simulink model "simRouteA_v4_11"  (R2015a)
settings: Solver=FixedStepDiscrete  StartTime=0.0  StopTime=36000  FixedStep=1  RelTol=1e-3
PreLoadFcn:
  | loadTimetable
StopFcn:
  | postProcess
undefined symbols (not defined in the file or in its folder): setBus1IntergenTime, setBus2IntergenTime, setBus3IntergenTime, setBus4IntergenTime
(part 2 of 7)

== system simRouteA_v4_11/Subsystem ==
  ID : Inport
  tTable : Inport  Port=2
  Constant12 : Constant  Value=10000
  Constant13 : Constant
  Direct Lookup Table (n-D)1 : LookupNDDirect  TableIsInput=on
  Divide1 : Product  Inputs=/*
  Math Function1 : Math  Operator=mod  SaturateOnIntegerOverflow=on
  Rounding : Rounding  Operator=round
  Rounding1 : Rounding  Operator=round
  Subtract1 : Sum  Inputs=-+
  schedTime : Outport
  wires:
  Rounding1/1 -> Direct Lookup Table (n-D)1/1
  Constant12/1 -> Math Function1/2, Divide1/1
  Constant13/1 -> Subtract1/1
  Divide1/1 -> Rounding/1
  Subtract1/1 -> Direct Lookup Table (n-D)1/2
  Direct Lookup Table (n-D)1/1 -> schedTime/1
  tTable/1 -> Direct Lookup Table (n-D)1/3
  Math Function1/1 -> Rounding1/1
  Rounding/1 -> Subtract1/2
  ID/1 -> Divide1/2, Math Function1/1

== system simRouteA_v4_11/Subsystem3 ==
  crnSched : Inport
  time : Inport  Port=2
  Constant2 : Constant  Value=0
  MinMax : MinMax  Function=max  Inputs=2
  Subtract1 : Sum  Inputs=+-
  tHoldCrnBus : Outport
  wires:
  time/1 -> Subtract1/2
  crnSched/1 -> Subtract1/1
  Subtract1/1 -> MinMax/1
  MinMax/1 -> tHoldCrnBus/1
  Constant2/1 -> MinMax/2

== system simRouteA_v4_11/atStopS1 ==
  paxDemandRate : Inport
  paxAlightRate : Inport  Port=2
  FIFO Queue9 : FIFOQueue
  busDwellThisStop : Subsystem
  calcPaxActivThisStop : Subsystem
  integrPaxAlightS1 : Subsystem
  integrPaxArrS1 : Subsystem
  setPaxAttribThisStop : SetAttribute  AttributeName=paxArr|paxAlight  AttributeFrom=Signal port|Signal port  AttributeValue=1|1  AttributeTreatAsVector=1|1  EvaluatedAttributeValue={ []; [] }
      settings: InputPortMap=u0,u1
  busIn : PMIOPort  Port=1  Side=Left
  busOut : PMIOPort  Port=2  Side=Right
  accPaxAlight : Outport
  accPaxDemand : Outport  Port=2
  crnVacancy : Outport  Port=3
  paxAlight : Outport  Port=4
  paxDemand : Outport  Port=5
  busIDAfterPaxCal : Outport  Port=6
  newVacancy : Outport  Port=7
  paxBoard : Outport  Port=8
  paxRemain : Outport  Port=9
  paxWait : Outport  Port=10
  intgPaxArr : Outport  Port=11
  intgPaxAlight : Outport  Port=12
  idBusLeave : Outport  Port=13
  wires:
  calcPaxActivThisStop/4(busID) -> busIDAfterPaxCal/1
  calcPaxActivThisStop/1(vacanIn) -> crnVacancy/1
  calcPaxActivThisStop/5(newVacan) -> newVacancy/1
  calcPaxActivThisStop/7(paxRemain) -> paxRemain/1
  paxAlightRate/1 -> integrPaxAlightS1/1(ratePax)
  calcPaxActivThisStop/3(paxArr) -> paxDemand/1
  busDwellThisStop/1(idBusLeave) -> idBusLeave/1
  calcPaxActivThisStop/6(paxBoard) -> paxBoard/1
  calcPaxActivThisStop/9(intgPaxArr) -> intgPaxArr/1
  calcPaxActivThisStop/8(paxWait) -> paxWait/1
  integrPaxArrS1/1(accPax) -> accPaxDemand/1, setPaxAttribThisStop/1
  integrPaxAlightS1/1(accPax) -> accPaxAlight/1, setPaxAttribThisStop/2
  calcPaxActivThisStop/11(dwellTime) -> busDwellThisStop/1(dwellTime)
  calcPaxActivThisStop/10(intgPaxAlight) -> intgPaxAlight/1
  calcPaxActivThisStop/2(paxAlight) -> paxAlight/1
  paxDemandRate/1 -> integrPaxArrS1/1(ratePax)
  connections:
  FIFO Queue9/LConn1 -- busIn/RConn1
  busDwellThisStop/RConn1 -- busOut/RConn1
  setPaxAttribThisStop/RConn1 -- calcPaxActivThisStop/LConn1
  FIFO Queue9/RConn1 -- setPaxAttribThisStop/LConn1
  busDwellThisStop/LConn1 -- calcPaxActivThisStop/RConn1

== system simRouteA_v4_11/atStopS10 ==
  paxDemandRate : Inport
  paxAlightRate : Inport  Port=2
  FIFO Queue9 : FIFOQueue
  busDwellThisStop : Subsystem
  calcPaxActivThisStop : Subsystem
  integrPaxAlightS1 : Subsystem
  integrPaxArrS1 : Subsystem
  setPaxAttribThisStop : SetAttribute  AttributeName=paxArr|paxAlight  AttributeFrom=Signal port|Signal port  AttributeValue=1|1  AttributeTreatAsVector=1|1  EvaluatedAttributeValue={ []; [] }
      settings: InputPortMap=u0,u1
  busIn : PMIOPort  Port=1  Side=Left
  busOut : PMIOPort  Port=2  Side=Right
  accPaxAlight : Outport
  accPaxDemand : Outport  Port=2
  crnVacancy : Outport  Port=3
  paxAlight : Outport  Port=4
  paxDemand : Outport  Port=5
  busIDAfterPaxCal : Outport  Port=6
  newVacancy : Outport  Port=7
  paxBoard : Outport  Port=8
  paxRemain : Outport  Port=9
  paxWait : Outport  Port=10
  intgPaxArr : Outport  Port=11
  intgPaxAlight : Outport  Port=12
  idBusLeave : Outport  Port=13
  wires:
  calcPaxActivThisStop/4(busID) -> busIDAfterPaxCal/1
  calcPaxActivThisStop/1(vacanIn) -> crnVacancy/1
  calcPaxActivThisStop/5(newVacan) -> newVacancy/1
  calcPaxActivThisStop/7(paxRemain) -> paxRemain/1
  paxAlightRate/1 -> integrPaxAlightS1/1(ratePax)
  calcPaxActivThisStop/3(paxArr) -> paxDemand/1
  busDwellThisStop/1(idBusLeave) -> idBusLeave/1
  calcPaxActivThisStop/6(paxBoard) -> paxBoard/1
  calcPaxActivThisStop/9(intgPaxArr) -> intgPaxArr/1
  calcPaxActivThisStop/8(paxWait) -> paxWait/1
  integrPaxArrS1/1(accPax) -> accPaxDemand/1, setPaxAttribThisStop/1
  integrPaxAlightS1/1(accPax) -> accPaxAlight/1, setPaxAttribThisStop/2
  calcPaxActivThisStop/11(dwellTime) -> busDwellThisStop/1(dwellTime)
  calcPaxActivThisStop/10(intgPaxAlight) -> intgPaxAlight/1
  calcPaxActivThisStop/2(paxAlight) -> paxAlight/1
  paxDemandRate/1 -> integrPaxArrS1/1(ratePax)
  connections:
  FIFO Queue9/LConn1 -- busIn/RConn1
  busDwellThisStop/RConn1 -- busOut/RConn1
  setPaxAttribThisStop/RConn1 -- calcPaxActivThisStop/LConn1
  FIFO Queue9/RConn1 -- setPaxAttribThisStop/LConn1
  busDwellThisStop/LConn1 -- calcPaxActivThisStop/RConn1

== system simRouteA_v4_11/atStopS11 ==
  paxDemandRate : Inport
  paxAlightRate : Inport  Port=2
  FIFO Queue9 : FIFOQueue
  busDwellThisStop : Subsystem
  calcPaxActivThisStop : Subsystem
  integrPaxAlightS1 : Subsystem
  integrPaxArrS1 : Subsystem
  setPaxAttribThisStop : SetAttribute  AttributeName=paxArr|paxAlight  AttributeFrom=Signal port|Signal port  AttributeValue=1|1  AttributeTreatAsVector=1|1  EvaluatedAttributeValue={ []; [] }
      settings: InputPortMap=u0,u1
  busIn : PMIOPort  Port=1  Side=Left
  busOut : PMIOPort  Port=2  Side=Right
  accPaxAlight : Outport
  accPaxDemand : Outport  Port=2
  crnVacancy : Outport  Port=3
  paxAlight : Outport  Port=4
  paxDemand : Outport  Port=5
  busIDAfterPaxCal : Outport  Port=6
  newVacancy : Outport  Port=7
  paxBoard : Outport  Port=8
  paxRemain : Outport  Port=9
  paxWait : Outport  Port=10
  intgPaxArr : Outport  Port=11
  intgPaxAlight : Outport  Port=12
  idBusLeave : Outport  Port=13
  wires:
  calcPaxActivThisStop/4(busID) -> busIDAfterPaxCal/1
  calcPaxActivThisStop/1(vacanIn) -> crnVacancy/1
  calcPaxActivThisStop/5(newVacan) -> newVacancy/1
  calcPaxActivThisStop/7(paxRemain) -> paxRemain/1
  paxAlightRate/1 -> integrPaxAlightS1/1(ratePax)
  calcPaxActivThisStop/3(paxArr) -> paxDemand/1
  busDwellThisStop/1(idBusLeave) -> idBusLeave/1
  calcPaxActivThisStop/6(paxBoard) -> paxBoard/1
  calcPaxActivThisStop/9(intgPaxArr) -> intgPaxArr/1
  calcPaxActivThisStop/8(paxWait) -> paxWait/1
  integrPaxArrS1/1(accPax) -> accPaxDemand/1, setPaxAttribThisStop/1
  integrPaxAlightS1/1(accPax) -> accPaxAlight/1, setPaxAttribThisStop/2
  calcPaxActivThisStop/11(dwellTime) -> busDwellThisStop/1(dwellTime)
  calcPaxActivThisStop/10(intgPaxAlight) -> intgPaxAlight/1
  calcPaxActivThisStop/2(paxAlight) -> paxAlight/1
  paxDemandRate/1 -> integrPaxArrS1/1(ratePax)
  connections:
  FIFO Queue9/LConn1 -- busIn/RConn1
  busDwellThisStop/RConn1 -- busOut/RConn1
  setPaxAttribThisStop/RConn1 -- calcPaxActivThisStop/LConn1
  FIFO Queue9/RConn1 -- setPaxAttribThisStop/LConn1
  busDwellThisStop/LConn1 -- calcPaxActivThisStop/RConn1

== system simRouteA_v4_11/atStopS12 ==
  paxDemandRate : Inport
  paxAlightRate : Inport  Port=2
  FIFO Queue9 : FIFOQueue
  busDwellThisStop : Subsystem
  calcPaxActivThisStop : Subsystem
  integrPaxAlightS1 : Subsystem
  integrPaxArrS1 : Subsystem
  setPaxAttribThisStop : SetAttribute  AttributeName=paxArr|paxAlight  AttributeFrom=Signal port|Signal port  AttributeValue=1|1  AttributeTreatAsVector=1|1  EvaluatedAttributeValue={ []; [] }
      settings: InputPortMap=u0,u1
  busIn : PMIOPort  Port=1  Side=Left
  busOut : PMIOPort  Port=2  Side=Right
  accPaxAlight : Outport
  accPaxDemand : Outport  Port=2
  crnVacancy : Outport  Port=3
  paxAlight : Outport  Port=4
  paxDemand : Outport  Port=5
  busIDAfterPaxCal : Outport  Port=6
  newVacancy : Outport  Port=7
  paxBoard : Outport  Port=8
  paxRemain : Outport  Port=9
  paxWait : Outport  Port=10
  intgPaxArr : Outport  Port=11
  intgPaxAlight : Outport  Port=12
  idBusLeave : Outport  Port=13
  wires:
  calcPaxActivThisStop/4(busID) -> busIDAfterPaxCal/1
  calcPaxActivThisStop/1(vacanIn) -> crnVacancy/1
  calcPaxActivThisStop/5(newVacan) -> newVacancy/1
  calcPaxActivThisStop/7(paxRemain) -> paxRemain/1
  paxAlightRate/1 -> integrPaxAlightS1/1(ratePax)
  calcPaxActivThisStop/3(paxArr) -> paxDemand/1
  busDwellThisStop/1(idBusLeave) -> idBusLeave/1
  calcPaxActivThisStop/6(paxBoard) -> paxBoard/1
  calcPaxActivThisStop/9(intgPaxArr) -> intgPaxArr/1
  calcPaxActivThisStop/8(paxWait) -> paxWait/1
  integrPaxArrS1/1(accPax) -> accPaxDemand/1, setPaxAttribThisStop/1
  integrPaxAlightS1/1(accPax) -> accPaxAlight/1, setPaxAttribThisStop/2
  calcPaxActivThisStop/11(dwellTime) -> busDwellThisStop/1(dwellTime)
  calcPaxActivThisStop/10(intgPaxAlight) -> intgPaxAlight/1
  calcPaxActivThisStop/2(paxAlight) -> paxAlight/1
  paxDemandRate/1 -> integrPaxArrS1/1(ratePax)
  connections:
  FIFO Queue9/LConn1 -- busIn/RConn1
  busDwellThisStop/RConn1 -- busOut/RConn1
  setPaxAttribThisStop/RConn1 -- calcPaxActivThisStop/LConn1
  FIFO Queue9/RConn1 -- setPaxAttribThisStop/LConn1
  busDwellThisStop/LConn1 -- calcPaxActivThisStop/RConn1

== system simRouteA_v4_11/atStopS13 ==
  paxDemandRate : Inport
  paxAlightRate : Inport  Port=2
  FIFO Queue9 : FIFOQueue
  busDwellThisStop : Subsystem
  calcPaxActivThisStop : Subsystem
  integrPaxAlightS1 : Subsystem
  integrPaxArrS1 : Subsystem
  setPaxAttribThisStop : SetAttribute  AttributeName=paxArr|paxAlight  AttributeFrom=Signal port|Signal port  AttributeValue=1|1  AttributeTreatAsVector=1|1  EvaluatedAttributeValue={ []; [] }
      settings: InputPortMap=u0,u1
  busIn : PMIOPort  Port=1  Side=Left
  busOut : PMIOPort  Port=2  Side=Right
  accPaxAlight : Outport
  accPaxDemand : Outport  Port=2
  crnVacancy : Outport  Port=3
  paxAlight : Outport  Port=4
  paxDemand : Outport  Port=5
  busIDAfterPaxCal : Outport  Port=6
  newVacancy : Outport  Port=7
  paxBoard : Outport  Port=8
  paxRemain : Outport  Port=9
  paxWait : Outport  Port=10
  intgPaxArr : Outport  Port=11
  intgPaxAlight : Outport  Port=12
  idBusLeave : Outport  Port=13
  wires:
  calcPaxActivThisStop/4(busID) -> busIDAfterPaxCal/1
  calcPaxActivThisStop/1(vacanIn) -> crnVacancy/1
  calcPaxActivThisStop/5(newVacan) -> newVacancy/1
  calcPaxActivThisStop/7(paxRemain) -> paxRemain/1
  paxAlightRate/1 -> integrPaxAlightS1/1(ratePax)
  calcPaxActivThisStop/3(paxArr) -> paxDemand/1
  busDwellThisStop/1(idBusLeave) -> idBusLeave/1
  calcPaxActivThisStop/6(paxBoard) -> paxBoard/1
  calcPaxActivThisStop/9(intgPaxArr) -> intgPaxArr/1
  calcPaxActivThisStop/8(paxWait) -> paxWait/1
  integrPaxArrS1/1(accPax) -> accPaxDemand/1, setPaxAttribThisStop/1
  integrPaxAlightS1/1(accPax) -> accPaxAlight/1, setPaxAttribThisStop/2
  calcPaxActivThisStop/11(dwellTime) -> busDwellThisStop/1(dwellTime)
  calcPaxActivThisStop/10(intgPaxAlight) -> intgPaxAlight/1
  calcPaxActivThisStop/2(paxAlight) -> paxAlight/1
  paxDemandRate/1 -> integrPaxArrS1/1(ratePax)
  connections:
  FIFO Queue9/LConn1 -- busIn/RConn1
  busDwellThisStop/RConn1 -- busOut/RConn1
  setPaxAttribThisStop/RConn1 -- calcPaxActivThisStop/LConn1
  FIFO Queue9/RConn1 -- setPaxAttribThisStop/LConn1
  busDwellThisStop/LConn1 -- calcPaxActivThisStop/RConn1

== system simRouteA_v4_11/atStopS14 ==
  paxDemandRate : Inport
  paxAlightRate : Inport  Port=2
  FIFO Queue9 : FIFOQueue
  busDwellThisStop : Subsystem
  calcPaxActivThisStop : Subsystem
  integrPaxAlightS1 : Subsystem
  integrPaxArrS1 : Subsystem
  setPaxAttribThisStop : SetAttribute  AttributeName=paxArr|paxAlight  AttributeFrom=Signal port|Signal port  AttributeValue=1|1  AttributeTreatAsVector=1|1  EvaluatedAttributeValue={ []; [] }
      settings: InputPortMap=u0,u1
  busIn : PMIOPort  Port=1  Side=Left
  busOut : PMIOPort  Port=2  Side=Right
  accPaxAlight : Outport
  accPaxDemand : Outport  Port=2
  crnVacancy : Outport  Port=3
  paxAlight : Outport  Port=4
  paxDemand : Outport  Port=5
  busIDAfterPaxCal : Outport  Port=6
  newVacancy : Outport  Port=7
  paxBoard : Outport  Port=8
  paxRemain : Outport  Port=9
  paxWait : Outport  Port=10
  intgPaxArr : Outport  Port=11
  intgPaxAlight : Outport  Port=12
  idBusLeave : Outport  Port=13
  wires:
  calcPaxActivThisStop/4(busID) -> busIDAfterPaxCal/1
  calcPaxActivThisStop/1(vacanIn) -> crnVacancy/1
  calcPaxActivThisStop/5(newVacan) -> newVacancy/1
  calcPaxActivThisStop/7(paxRemain) -> paxRemain/1
  paxAlightRate/1 -> integrPaxAlightS1/1(ratePax)
  calcPaxActivThisStop/3(paxArr) -> paxDemand/1
  busDwellThisStop/1(idBusLeave) -> idBusLeave/1
  calcPaxActivThisStop/6(paxBoard) -> paxBoard/1
  calcPaxActivThisStop/9(intgPaxArr) -> intgPaxArr/1
  calcPaxActivThisStop/8(paxWait) -> paxWait/1
  integrPaxArrS1/1(accPax) -> accPaxDemand/1, setPaxAttribThisStop/1
  integrPaxAlightS1/1(accPax) -> accPaxAlight/1, setPaxAttribThisStop/2
  calcPaxActivThisStop/11(dwellTime) -> busDwellThisStop/1(dwellTime)
  calcPaxActivThisStop/10(intgPaxAlight) -> intgPaxAlight/1
  calcPaxActivThisStop/2(paxAlight) -> paxAlight/1
  paxDemandRate/1 -> integrPaxArrS1/1(ratePax)
  connections:
  FIFO Queue9/LConn1 -- busIn/RConn1
  busDwellThisStop/RConn1 -- busOut/RConn1
  setPaxAttribThisStop/RConn1 -- calcPaxActivThisStop/LConn1
  FIFO Queue9/RConn1 -- setPaxAttribThisStop/LConn1
  busDwellThisStop/LConn1 -- calcPaxActivThisStop/RConn1

== system simRouteA_v4_11/atStopS15 ==
  paxDemandRate : Inport
  paxAlightRate : Inport  Port=2
  FIFO Queue9 : FIFOQueue
  busDwellThisStop : Subsystem
  calcPaxActivThisStop : Subsystem
  integrPaxAlightS1 : Subsystem
  integrPaxArrS1 : Subsystem
  setPaxAttribThisStop : SetAttribute  AttributeName=paxArr|paxAlight  AttributeFrom=Signal port|Signal port  AttributeValue=1|1  AttributeTreatAsVector=1|1  EvaluatedAttributeValue={ []; [] }
      settings: InputPortMap=u0,u1
  busIn : PMIOPort  Port=1  Side=Left
  busOut : PMIOPort  Port=2  Side=Right
  accPaxAlight : Outport
  accPaxDemand : Outport  Port=2
  crnVacancy : Outport  Port=3
  paxAlight : Outport  Port=4
  paxDemand : Outport  Port=5
  busIDAfterPaxCal : Outport  Port=6
  newVacancy : Outport  Port=7
  paxBoard : Outport  Port=8
  paxRemain : Outport  Port=9
  paxWait : Outport  Port=10
  intgPaxArr : Outport  Port=11
  intgPaxAlight : Outport  Port=12
  idBusLeave : Outport  Port=13
  wires:
  calcPaxActivThisStop/4(busID) -> busIDAfterPaxCal/1
  calcPaxActivThisStop/1(vacanIn) -> crnVacancy/1
  calcPaxActivThisStop/5(newVacan) -> newVacancy/1
  calcPaxActivThisStop/7(paxRemain) -> paxRemain/1
  paxAlightRate/1 -> integrPaxAlightS1/1(ratePax)
  calcPaxActivThisStop/3(paxArr) -> paxDemand/1
  busDwellThisStop/1(idBusLeave) -> idBusLeave/1
  calcPaxActivThisStop/6(paxBoard) -> paxBoard/1
  calcPaxActivThisStop/9(intgPaxArr) -> intgPaxArr/1
  calcPaxActivThisStop/8(paxWait) -> paxWait/1
  integrPaxArrS1/1(accPax) -> accPaxDemand/1, setPaxAttribThisStop/1
  integrPaxAlightS1/1(accPax) -> accPaxAlight/1, setPaxAttribThisStop/2
  calcPaxActivThisStop/11(dwellTime) -> busDwellThisStop/1(dwellTime)
  calcPaxActivThisStop/10(intgPaxAlight) -> intgPaxAlight/1
  calcPaxActivThisStop/2(paxAlight) -> paxAlight/1
  paxDemandRate/1 -> integrPaxArrS1/1(ratePax)
  connections:
  FIFO Queue9/LConn1 -- busIn/RConn1
  busDwellThisStop/RConn1 -- busOut/RConn1
  setPaxAttribThisStop/RConn1 -- calcPaxActivThisStop/LConn1
  FIFO Queue9/RConn1 -- setPaxAttribThisStop/LConn1
  busDwellThisStop/LConn1 -- calcPaxActivThisStop/RConn1

== system simRouteA_v4_11/atStopS16 ==
  paxDemandRate : Inport
  paxAlightRate : Inport  Port=2
  FIFO Queue9 : FIFOQueue
  busDwellThisStop : Subsystem
  calcPaxActivThisStop : Subsystem
  integrPaxAlightS1 : Subsystem
  integrPaxArrS1 : Subsystem
  setPaxAttribThisStop : SetAttribute  AttributeName=paxArr|paxAlight  AttributeFrom=Signal port|Signal port  AttributeValue=1|1  AttributeTreatAsVector=1|1  EvaluatedAttributeValue={ []; [] }
      settings: InputPortMap=u0,u1
  busIn : PMIOPort  Port=1  Side=Left
  busOut : PMIOPort  Port=2  Side=Right
  accPaxAlight : Outport
  accPaxDemand : Outport  Port=2
  crnVacancy : Outport  Port=3
  paxAlight : Outport  Port=4
  paxDemand : Outport  Port=5
  busIDAfterPaxCal : Outport  Port=6
  newVacancy : Outport  Port=7
  paxBoard : Outport  Port=8
  paxRemain : Outport  Port=9
  paxWait : Outport  Port=10
  intgPaxArr : Outport  Port=11
  intgPaxAlight : Outport  Port=12
  idBusLeave : Outport  Port=13
  wires:
  calcPaxActivThisStop/4(busID) -> busIDAfterPaxCal/1
  calcPaxActivThisStop/1(vacanIn) -> crnVacancy/1
  calcPaxActivThisStop/5(newVacan) -> newVacancy/1
  calcPaxActivThisStop/7(paxRemain) -> paxRemain/1
  paxAlightRate/1 -> integrPaxAlightS1/1(ratePax)
  calcPaxActivThisStop/3(paxArr) -> paxDemand/1
  busDwellThisStop/1(idBusLeave) -> idBusLeave/1
  calcPaxActivThisStop/6(paxBoard) -> paxBoard/1
  calcPaxActivThisStop/9(intgPaxArr) -> intgPaxArr/1
  calcPaxActivThisStop/8(paxWait) -> paxWait/1
  integrPaxArrS1/1(accPax) -> accPaxDemand/1, setPaxAttribThisStop/1
  integrPaxAlightS1/1(accPax) -> accPaxAlight/1, setPaxAttribThisStop/2
  calcPaxActivThisStop/11(dwellTime) -> busDwellThisStop/1(dwellTime)
  calcPaxActivThisStop/10(intgPaxAlight) -> intgPaxAlight/1
  calcPaxActivThisStop/2(paxAlight) -> paxAlight/1
  paxDemandRate/1 -> integrPaxArrS1/1(ratePax)
  connections:
  FIFO Queue9/LConn1 -- busIn/RConn1
  busDwellThisStop/RConn1 -- busOut/RConn1
  setPaxAttribThisStop/RConn1 -- calcPaxActivThisStop/LConn1
  FIFO Queue9/RConn1 -- setPaxAttribThisStop/LConn1
  busDwellThisStop/LConn1 -- calcPaxActivThisStop/RConn1

== system simRouteA_v4_11/atStopS17 ==
  paxDemandRate : Inport
  paxAlightRate : Inport  Port=2
  FIFO Queue9 : FIFOQueue
  busDwellThisStop : Subsystem
  calcPaxActivThisStop : Subsystem
  integrPaxAlightS1 : Subsystem
  integrPaxArrS1 : Subsystem
  setPaxAttribThisStop : SetAttribute  AttributeName=paxArr|paxAlight  AttributeFrom=Signal port|Signal port  AttributeValue=1|1  AttributeTreatAsVector=1|1  EvaluatedAttributeValue={ []; [] }
      settings: InputPortMap=u0,u1
  busIn : PMIOPort  Port=1  Side=Left
  busOut : PMIOPort  Port=2  Side=Right
  accPaxAlight : Outport
  accPaxDemand : Outport  Port=2
  crnVacancy : Outport  Port=3
  paxAlight : Outport  Port=4
  paxDemand : Outport  Port=5
  busIDAfterPaxCal : Outport  Port=6
  newVacancy : Outport  Port=7
  paxBoard : Outport  Port=8
  paxRemain : Outport  Port=9
  paxWait : Outport  Port=10
  intgPaxArr : Outport  Port=11
  intgPaxAlight : Outport  Port=12
  idBusLeave : Outport  Port=13
  wires:
  calcPaxActivThisStop/4(busID) -> busIDAfterPaxCal/1
  calcPaxActivThisStop/1(vacanIn) -> crnVacancy/1
  calcPaxActivThisStop/5(newVacan) -> newVacancy/1
  calcPaxActivThisStop/7(paxRemain) -> paxRemain/1
  paxAlightRate/1 -> integrPaxAlightS1/1(ratePax)
  calcPaxActivThisStop/3(paxArr) -> paxDemand/1
  busDwellThisStop/1(idBusLeave) -> idBusLeave/1
  calcPaxActivThisStop/6(paxBoard) -> paxBoard/1
  calcPaxActivThisStop/9(intgPaxArr) -> intgPaxArr/1
  calcPaxActivThisStop/8(paxWait) -> paxWait/1
  integrPaxArrS1/1(accPax) -> accPaxDemand/1, setPaxAttribThisStop/1
  integrPaxAlightS1/1(accPax) -> accPaxAlight/1, setPaxAttribThisStop/2
  calcPaxActivThisStop/11(dwellTime) -> busDwellThisStop/1(dwellTime)
  calcPaxActivThisStop/10(intgPaxAlight) -> intgPaxAlight/1
  calcPaxActivThisStop/2(paxAlight) -> paxAlight/1
  paxDemandRate/1 -> integrPaxArrS1/1(ratePax)
  connections:
  FIFO Queue9/LConn1 -- busIn/RConn1
  busDwellThisStop/RConn1 -- busOut/RConn1
  setPaxAttribThisStop/RConn1 -- calcPaxActivThisStop/LConn1
  FIFO Queue9/RConn1 -- setPaxAttribThisStop/LConn1
  busDwellThisStop/LConn1 -- calcPaxActivThisStop/RConn1

== system simRouteA_v4_11/atStopS18 ==
  paxDemandRate : Inport
  paxAlightRate : Inport  Port=2
  FIFO Queue9 : FIFOQueue
  busDwellThisStop : Subsystem
  calcPaxActivThisStop : Subsystem
  integrPaxAlightS1 : Subsystem
  integrPaxArrS1 : Subsystem
  setPaxAttribThisStop : SetAttribute  AttributeName=paxArr|paxAlight  AttributeFrom=Signal port|Signal port  AttributeValue=1|1  AttributeTreatAsVector=1|1  EvaluatedAttributeValue={ []; [] }
      settings: InputPortMap=u0,u1
  busIn : PMIOPort  Port=1  Side=Left
  busOut : PMIOPort  Port=2  Side=Right
  accPaxAlight : Outport
  accPaxDemand : Outport  Port=2
  crnVacancy : Outport  Port=3
  paxAlight : Outport  Port=4
  paxDemand : Outport  Port=5
  busIDAfterPaxCal : Outport  Port=6
  newVacancy : Outport  Port=7
  paxBoard : Outport  Port=8
  paxRemain : Outport  Port=9
  paxWait : Outport  Port=10
  intgPaxArr : Outport  Port=11
  intgPaxAlight : Outport  Port=12
  idBusLeave : Outport  Port=13
  wires:
  calcPaxActivThisStop/4(busID) -> busIDAfterPaxCal/1
  calcPaxActivThisStop/1(vacanIn) -> crnVacancy/1
  calcPaxActivThisStop/5(newVacan) -> newVacancy/1
  calcPaxActivThisStop/7(paxRemain) -> paxRemain/1
  paxAlightRate/1 -> integrPaxAlightS1/1(ratePax)
  calcPaxActivThisStop/3(paxArr) -> paxDemand/1
  busDwellThisStop/1(idBusLeave) -> idBusLeave/1
  calcPaxActivThisStop/6(paxBoard) -> paxBoard/1
  calcPaxActivThisStop/9(intgPaxArr) -> intgPaxArr/1
  calcPaxActivThisStop/8(paxWait) -> paxWait/1
  integrPaxArrS1/1(accPax) -> accPaxDemand/1, setPaxAttribThisStop/1
  integrPaxAlightS1/1(accPax) -> accPaxAlight/1, setPaxAttribThisStop/2
  calcPaxActivThisStop/11(dwellTime) -> busDwellThisStop/1(dwellTime)
  calcPaxActivThisStop/10(intgPaxAlight) -> intgPaxAlight/1
  calcPaxActivThisStop/2(paxAlight) -> paxAlight/1
  paxDemandRate/1 -> integrPaxArrS1/1(ratePax)
  connections:
  FIFO Queue9/LConn1 -- busIn/RConn1
  busDwellThisStop/RConn1 -- busOut/RConn1
  setPaxAttribThisStop/RConn1 -- calcPaxActivThisStop/LConn1
  FIFO Queue9/RConn1 -- setPaxAttribThisStop/LConn1
  busDwellThisStop/LConn1 -- calcPaxActivThisStop/RConn1

== system simRouteA_v4_11/atStopS2 ==
  paxDemandRate : Inport
  paxAlightRate : Inport  Port=2
  FIFO Queue9 : FIFOQueue
  busDwellThisStop : Subsystem
  calcPaxActivThisStop : Subsystem
  integrPaxAlightS1 : Subsystem
  integrPaxArrS1 : Subsystem
  setPaxAttribThisStop : SetAttribute  AttributeName=paxArr|paxAlight  AttributeFrom=Signal port|Signal port  AttributeValue=1|1  AttributeTreatAsVector=1|1  EvaluatedAttributeValue={ []; [] }
      settings: InputPortMap=u0,u1
  busIn : PMIOPort  Port=1  Side=Left
  busOut : PMIOPort  Port=2  Side=Right
  accPaxAlight : Outport
  accPaxDemand : Outport  Port=2
  crnVacancy : Outport  Port=3
  paxAlight : Outport  Port=4
  paxDemand : Outport  Port=5
  busIDAfterPaxCal : Outport  Port=6
  newVacancy : Outport  Port=7
  paxBoard : Outport  Port=8
  paxRemain : Outport  Port=9
  paxWait : Outport  Port=10
  intgPaxArr : Outport  Port=11
  intgPaxAlight : Outport  Port=12
  idBusLeave : Outport  Port=13
  wires:
  calcPaxActivThisStop/4(busID) -> busIDAfterPaxCal/1
  calcPaxActivThisStop/1(vacanIn) -> crnVacancy/1
  calcPaxActivThisStop/5(newVacan) -> newVacancy/1
  calcPaxActivThisStop/7(paxRemain) -> paxRemain/1
  paxAlightRate/1 -> integrPaxAlightS1/1(ratePax)
  calcPaxActivThisStop/3(paxArr) -> paxDemand/1
  busDwellThisStop/1(idBusLeave) -> idBusLeave/1
  calcPaxActivThisStop/6(paxBoard) -> paxBoard/1
  calcPaxActivThisStop/9(intgPaxArr) -> intgPaxArr/1
  calcPaxActivThisStop/8(paxWait) -> paxWait/1
  integrPaxArrS1/1(accPax) -> accPaxDemand/1, setPaxAttribThisStop/1
  integrPaxAlightS1/1(accPax) -> accPaxAlight/1, setPaxAttribThisStop/2
  calcPaxActivThisStop/11(dwellTime) -> busDwellThisStop/1(dwellTime)
  calcPaxActivThisStop/10(intgPaxAlight) -> intgPaxAlight/1
  calcPaxActivThisStop/2(paxAlight) -> paxAlight/1
  paxDemandRate/1 -> integrPaxArrS1/1(ratePax)
  connections:
  FIFO Queue9/LConn1 -- busIn/RConn1
  busDwellThisStop/RConn1 -- busOut/RConn1
  setPaxAttribThisStop/RConn1 -- calcPaxActivThisStop/LConn1
  FIFO Queue9/RConn1 -- setPaxAttribThisStop/LConn1
  busDwellThisStop/LConn1 -- calcPaxActivThisStop/RConn1

== system simRouteA_v4_11/atStopS3 ==
  paxDemandRate : Inport
  paxAlightRate : Inport  Port=2
  FIFO Queue9 : FIFOQueue
  busDwellThisStop : Subsystem
  calcPaxActivThisStop : Subsystem
  integrPaxAlightS1 : Subsystem
  integrPaxArrS1 : Subsystem
  setPaxAttribThisStop : SetAttribute  AttributeName=paxArr|paxAlight  AttributeFrom=Signal port|Signal port  AttributeValue=1|1  AttributeTreatAsVector=1|1  EvaluatedAttributeValue={ []; [] }
      settings: InputPortMap=u0,u1
  busIn : PMIOPort  Port=1  Side=Left
  busOut : PMIOPort  Port=2  Side=Right
  accPaxAlight : Outport
  accPaxDemand : Outport  Port=2
  crnVacancy : Outport  Port=3
  paxAlight : Outport  Port=4
  paxDemand : Outport  Port=5
  busIDAfterPaxCal : Outport  Port=6
  newVacancy : Outport  Port=7
  paxBoard : Outport  Port=8
  paxRemain : Outport  Port=9
  paxWait : Outport  Port=10
  intgPaxArr : Outport  Port=11
  intgPaxAlight : Outport  Port=12
  idBusLeave : Outport  Port=13
  wires:
  calcPaxActivThisStop/4(busID) -> busIDAfterPaxCal/1
  calcPaxActivThisStop/1(vacanIn) -> crnVacancy/1
  calcPaxActivThisStop/5(newVacan) -> newVacancy/1
  calcPaxActivThisStop/7(paxRemain) -> paxRemain/1
  paxAlightRate/1 -> integrPaxAlightS1/1(ratePax)
  calcPaxActivThisStop/3(paxArr) -> paxDemand/1
  busDwellThisStop/1(idBusLeave) -> idBusLeave/1
  calcPaxActivThisStop/6(paxBoard) -> paxBoard/1
  calcPaxActivThisStop/9(intgPaxArr) -> intgPaxArr/1
  calcPaxActivThisStop/8(paxWait) -> paxWait/1
  integrPaxArrS1/1(accPax) -> accPaxDemand/1, setPaxAttribThisStop/1
  integrPaxAlightS1/1(accPax) -> accPaxAlight/1, setPaxAttribThisStop/2
  calcPaxActivThisStop/11(dwellTime) -> busDwellThisStop/1(dwellTime)
  calcPaxActivThisStop/10(intgPaxAlight) -> intgPaxAlight/1
  calcPaxActivThisStop/2(paxAlight) -> paxAlight/1
  paxDemandRate/1 -> integrPaxArrS1/1(ratePax)
  connections:
  FIFO Queue9/LConn1 -- busIn/RConn1
  busDwellThisStop/RConn1 -- busOut/RConn1
  setPaxAttribThisStop/RConn1 -- calcPaxActivThisStop/LConn1
  FIFO Queue9/RConn1 -- setPaxAttribThisStop/LConn1
  busDwellThisStop/LConn1 -- calcPaxActivThisStop/RConn1

== system simRouteA_v4_11/atStopS4 ==
  paxDemandRate : Inport
  paxAlightRate : Inport  Port=2
  FIFO Queue9 : FIFOQueue
  busDwellThisStop : Subsystem
  calcPaxActivThisStop : Subsystem
  integrPaxAlightS1 : Subsystem
  integrPaxArrS1 : Subsystem
  setPaxAttribThisStop : SetAttribute  AttributeName=paxArr|paxAlight  AttributeFrom=Signal port|Signal port  AttributeValue=1|1  AttributeTreatAsVector=1|1  EvaluatedAttributeValue={ []; [] }
      settings: InputPortMap=u0,u1
  busIn : PMIOPort  Port=1  Side=Left
  busOut : PMIOPort  Port=2  Side=Right
  accPaxAlight : Outport
  accPaxDemand : Outport  Port=2
  crnVacancy : Outport  Port=3
  paxAlight : Outport  Port=4
  paxDemand : Outport  Port=5
  busIDAfterPaxCal : Outport  Port=6
  newVacancy : Outport  Port=7
  paxBoard : Outport  Port=8
  paxRemain : Outport  Port=9
  paxWait : Outport  Port=10
  intgPaxArr : Outport  Port=11
  intgPaxAlight : Outport  Port=12
  idBusLeave : Outport  Port=13
  wires:
  calcPaxActivThisStop/4(busID) -> busIDAfterPaxCal/1
  calcPaxActivThisStop/1(vacanIn) -> crnVacancy/1
  calcPaxActivThisStop/5(newVacan) -> newVacancy/1
  calcPaxActivThisStop/7(paxRemain) -> paxRemain/1
  paxAlightRate/1 -> integrPaxAlightS1/1(ratePax)
  calcPaxActivThisStop/3(paxArr) -> paxDemand/1
  busDwellThisStop/1(idBusLeave) -> idBusLeave/1
  calcPaxActivThisStop/6(paxBoard) -> paxBoard/1
  calcPaxActivThisStop/9(intgPaxArr) -> intgPaxArr/1
  calcPaxActivThisStop/8(paxWait) -> paxWait/1
  integrPaxArrS1/1(accPax) -> accPaxDemand/1, setPaxAttribThisStop/1
  integrPaxAlightS1/1(accPax) -> accPaxAlight/1, setPaxAttribThisStop/2
  calcPaxActivThisStop/11(dwellTime) -> busDwellThisStop/1(dwellTime)
  calcPaxActivThisStop/10(intgPaxAlight) -> intgPaxAlight/1
  calcPaxActivThisStop/2(paxAlight) -> paxAlight/1
  paxDemandRate/1 -> integrPaxArrS1/1(ratePax)
  connections:
  FIFO Queue9/LConn1 -- busIn/RConn1
  busDwellThisStop/RConn1 -- busOut/RConn1
  setPaxAttribThisStop/RConn1 -- calcPaxActivThisStop/LConn1
  FIFO Queue9/RConn1 -- setPaxAttribThisStop/LConn1
  busDwellThisStop/LConn1 -- calcPaxActivThisStop/RConn1

== system simRouteA_v4_11/atStopS5 ==
  paxDemandRate : Inport
  paxAlightRate : Inport  Port=2
  FIFO Queue9 : FIFOQueue
  busDwellThisStop : Subsystem
  calcPaxActivThisStop : Subsystem
  integrPaxAlightS1 : Subsystem
  integrPaxArrS1 : Subsystem
  setPaxAttribThisStop : SetAttribute  AttributeName=paxArr|paxAlight  AttributeFrom=Signal port|Signal port  AttributeValue=1|1  AttributeTreatAsVector=1|1  EvaluatedAttributeValue={ []; [] }
      settings: InputPortMap=u0,u1
  busIn : PMIOPort  Port=1  Side=Left
  busOut : PMIOPort  Port=2  Side=Right
  accPaxAlight : Outport
  accPaxDemand : Outport  Port=2
  crnVacancy : Outport  Port=3
  paxAlight : Outport  Port=4
  paxDemand : Outport  Port=5
  busIDAfterPaxCal : Outport  Port=6
  newVacancy : Outport  Port=7
  paxBoard : Outport  Port=8
  paxRemain : Outport  Port=9
  paxWait : Outport  Port=10
  intgPaxArr : Outport  Port=11
  intgPaxAlight : Outport  Port=12
  idBusLeave : Outport  Port=13
  wires:
  calcPaxActivThisStop/4(busID) -> busIDAfterPaxCal/1
  calcPaxActivThisStop/1(vacanIn) -> crnVacancy/1
  calcPaxActivThisStop/5(newVacan) -> newVacancy/1
  calcPaxActivThisStop/7(paxRemain) -> paxRemain/1
  paxAlightRate/1 -> integrPaxAlightS1/1(ratePax)
  calcPaxActivThisStop/3(paxArr) -> paxDemand/1
  busDwellThisStop/1(idBusLeave) -> idBusLeave/1
  calcPaxActivThisStop/6(paxBoard) -> paxBoard/1
  calcPaxActivThisStop/9(intgPaxArr) -> intgPaxArr/1
  calcPaxActivThisStop/8(paxWait) -> paxWait/1
  integrPaxArrS1/1(accPax) -> accPaxDemand/1, setPaxAttribThisStop/1
  integrPaxAlightS1/1(accPax) -> accPaxAlight/1, setPaxAttribThisStop/2
  calcPaxActivThisStop/11(dwellTime) -> busDwellThisStop/1(dwellTime)
  calcPaxActivThisStop/10(intgPaxAlight) -> intgPaxAlight/1
  calcPaxActivThisStop/2(paxAlight) -> paxAlight/1
  paxDemandRate/1 -> integrPaxArrS1/1(ratePax)
  connections:
  FIFO Queue9/LConn1 -- busIn/RConn1
  busDwellThisStop/RConn1 -- busOut/RConn1
  setPaxAttribThisStop/RConn1 -- calcPaxActivThisStop/LConn1
  FIFO Queue9/RConn1 -- setPaxAttribThisStop/LConn1
  busDwellThisStop/LConn1 -- calcPaxActivThisStop/RConn1

== system simRouteA_v4_11/atStopS6 ==
  paxDemandRate : Inport
  paxAlightRate : Inport  Port=2
  FIFO Queue9 : FIFOQueue
  busDwellThisStop : Subsystem
  calcPaxActivThisStop : Subsystem
  integrPaxAlightS1 : Subsystem
  integrPaxArrS1 : Subsystem
  setPaxAttribThisStop : SetAttribute  AttributeName=paxArr|paxAlight  AttributeFrom=Signal port|Signal port  AttributeValue=1|1  AttributeTreatAsVector=1|1  EvaluatedAttributeValue={ []; [] }
      settings: InputPortMap=u0,u1
  busIn : PMIOPort  Port=1  Side=Left
  busOut : PMIOPort  Port=2  Side=Right
  accPaxAlight : Outport
  accPaxDemand : Outport  Port=2
  crnVacancy : Outport  Port=3
  paxAlight : Outport  Port=4
  paxDemand : Outport  Port=5
  busIDAfterPaxCal : Outport  Port=6
  newVacancy : Outport  Port=7
  paxBoard : Outport  Port=8
  paxRemain : Outport  Port=9
  paxWait : Outport  Port=10
  intgPaxArr : Outport  Port=11
  intgPaxAlight : Outport  Port=12
  idBusLeave : Outport  Port=13
  wires:
  calcPaxActivThisStop/4(busID) -> busIDAfterPaxCal/1
  calcPaxActivThisStop/1(vacanIn) -> crnVacancy/1
  calcPaxActivThisStop/5(newVacan) -> newVacancy/1
  calcPaxActivThisStop/7(paxRemain) -> paxRemain/1
  paxAlightRate/1 -> integrPaxAlightS1/1(ratePax)
  calcPaxActivThisStop/3(paxArr) -> paxDemand/1
  busDwellThisStop/1(idBusLeave) -> idBusLeave/1
  calcPaxActivThisStop/6(paxBoard) -> paxBoard/1
  calcPaxActivThisStop/9(intgPaxArr) -> intgPaxArr/1
  calcPaxActivThisStop/8(paxWait) -> paxWait/1
  integrPaxArrS1/1(accPax) -> accPaxDemand/1, setPaxAttribThisStop/1
  integrPaxAlightS1/1(accPax) -> accPaxAlight/1, setPaxAttribThisStop/2
  calcPaxActivThisStop/11(dwellTime) -> busDwellThisStop/1(dwellTime)
  calcPaxActivThisStop/10(intgPaxAlight) -> intgPaxAlight/1
  calcPaxActivThisStop/2(paxAlight) -> paxAlight/1
  paxDemandRate/1 -> integrPaxArrS1/1(ratePax)
  connections:
  FIFO Queue9/LConn1 -- busIn/RConn1
  busDwellThisStop/RConn1 -- busOut/RConn1
  setPaxAttribThisStop/RConn1 -- calcPaxActivThisStop/LConn1
  FIFO Queue9/RConn1 -- setPaxAttribThisStop/LConn1
  busDwellThisStop/LConn1 -- calcPaxActivThisStop/RConn1

== system simRouteA_v4_11/atStopS7 ==
  paxDemandRate : Inport
  paxAlightRate : Inport  Port=2
  FIFO Queue9 : FIFOQueue
  busDwellThisStop : Subsystem
  calcPaxActivThisStop : Subsystem
  integrPaxAlightS1 : Subsystem
  integrPaxArrS1 : Subsystem
  setPaxAttribThisStop : SetAttribute  AttributeName=paxArr|paxAlight  AttributeFrom=Signal port|Signal port  AttributeValue=1|1  AttributeTreatAsVector=1|1  EvaluatedAttributeValue={ []; [] }
      settings: InputPortMap=u0,u1
  busIn : PMIOPort  Port=1  Side=Left
  busOut : PMIOPort  Port=2  Side=Right
  accPaxAlight : Outport
  accPaxDemand : Outport  Port=2
  crnVacancy : Outport  Port=3
  paxAlight : Outport  Port=4
  paxDemand : Outport  Port=5
  busIDAfterPaxCal : Outport  Port=6
  newVacancy : Outport  Port=7
  paxBoard : Outport  Port=8
  paxRemain : Outport  Port=9
  paxWait : Outport  Port=10
  intgPaxArr : Outport  Port=11
  intgPaxAlight : Outport  Port=12
  idBusLeave : Outport  Port=13
  wires:
  calcPaxActivThisStop/4(busID) -> busIDAfterPaxCal/1
  calcPaxActivThisStop/1(vacanIn) -> crnVacancy/1
  calcPaxActivThisStop/5(newVacan) -> newVacancy/1
  calcPaxActivThisStop/7(paxRemain) -> paxRemain/1
  paxAlightRate/1 -> integrPaxAlightS1/1(ratePax)
  calcPaxActivThisStop/3(paxArr) -> paxDemand/1
  busDwellThisStop/1(idBusLeave) -> idBusLeave/1
  calcPaxActivThisStop/6(paxBoard) -> paxBoard/1
  calcPaxActivThisStop/9(intgPaxArr) -> intgPaxArr/1
  calcPaxActivThisStop/8(paxWait) -> paxWait/1
  integrPaxArrS1/1(accPax) -> accPaxDemand/1, setPaxAttribThisStop/1
  integrPaxAlightS1/1(accPax) -> accPaxAlight/1, setPaxAttribThisStop/2
  calcPaxActivThisStop/11(dwellTime) -> busDwellThisStop/1(dwellTime)
  calcPaxActivThisStop/10(intgPaxAlight) -> intgPaxAlight/1
  calcPaxActivThisStop/2(paxAlight) -> paxAlight/1
  paxDemandRate/1 -> integrPaxArrS1/1(ratePax)
  connections:
  FIFO Queue9/LConn1 -- busIn/RConn1
  busDwellThisStop/RConn1 -- busOut/RConn1
  setPaxAttribThisStop/RConn1 -- calcPaxActivThisStop/LConn1
  FIFO Queue9/RConn1 -- setPaxAttribThisStop/LConn1
  busDwellThisStop/LConn1 -- calcPaxActivThisStop/RConn1

== system simRouteA_v4_11/atStopS8 ==
  paxDemandRate : Inport
  paxAlightRate : Inport  Port=2
  FIFO Queue9 : FIFOQueue
  busDwellThisStop : Subsystem
  calcPaxActivThisStop : Subsystem
  integrPaxAlightS1 : Subsystem
  integrPaxArrS1 : Subsystem
  setPaxAttribThisStop : SetAttribute  AttributeName=paxArr|paxAlight  AttributeFrom=Signal port|Signal port  AttributeValue=1|1  AttributeTreatAsVector=1|1  EvaluatedAttributeValue={ []; [] }
      settings: InputPortMap=u0,u1
  busIn : PMIOPort  Port=1  Side=Left
  busOut : PMIOPort  Port=2  Side=Right
  accPaxAlight : Outport
  accPaxDemand : Outport  Port=2
  crnVacancy : Outport  Port=3
  paxAlight : Outport  Port=4
  paxDemand : Outport  Port=5
  busIDAfterPaxCal : Outport  Port=6
  newVacancy : Outport  Port=7
  paxBoard : Outport  Port=8
  paxRemain : Outport  Port=9
  paxWait : Outport  Port=10
  intgPaxArr : Outport  Port=11
  intgPaxAlight : Outport  Port=12
  idBusLeave : Outport  Port=13
  wires:
  calcPaxActivThisStop/4(busID) -> busIDAfterPaxCal/1
  calcPaxActivThisStop/1(vacanIn) -> crnVacancy/1
  calcPaxActivThisStop/5(newVacan) -> newVacancy/1
  calcPaxActivThisStop/7(paxRemain) -> paxRemain/1
  paxAlightRate/1 -> integrPaxAlightS1/1(ratePax)
  calcPaxActivThisStop/3(paxArr) -> paxDemand/1
  busDwellThisStop/1(idBusLeave) -> idBusLeave/1
  calcPaxActivThisStop/6(paxBoard) -> paxBoard/1
  calcPaxActivThisStop/9(intgPaxArr) -> intgPaxArr/1
  calcPaxActivThisStop/8(paxWait) -> paxWait/1
  integrPaxArrS1/1(accPax) -> accPaxDemand/1, setPaxAttribThisStop/1
  integrPaxAlightS1/1(accPax) -> accPaxAlight/1, setPaxAttribThisStop/2
  calcPaxActivThisStop/11(dwellTime) -> busDwellThisStop/1(dwellTime)
  calcPaxActivThisStop/10(intgPaxAlight) -> intgPaxAlight/1
  calcPaxActivThisStop/2(paxAlight) -> paxAlight/1
  paxDemandRate/1 -> integrPaxArrS1/1(ratePax)
  connections:
  FIFO Queue9/LConn1 -- busIn/RConn1
  busDwellThisStop/RConn1 -- busOut/RConn1
  setPaxAttribThisStop/RConn1 -- calcPaxActivThisStop/LConn1
  FIFO Queue9/RConn1 -- setPaxAttribThisStop/LConn1
  busDwellThisStop/LConn1 -- calcPaxActivThisStop/RConn1

== system simRouteA_v4_11/atStopS9 ==
  paxDemandRate : Inport
  paxAlightRate : Inport  Port=2
  FIFO Queue9 : FIFOQueue
  busDwellThisStop : Subsystem
  calcPaxActivThisStop : Subsystem
  integrPaxAlightS1 : Subsystem
  integrPaxArrS1 : Subsystem
  setPaxAttribThisStop : SetAttribute  AttributeName=paxArr|paxAlight  AttributeFrom=Signal port|Signal port  AttributeValue=1|1  AttributeTreatAsVector=1|1  EvaluatedAttributeValue={ []; [] }
      settings: InputPortMap=u0,u1
  busIn : PMIOPort  Port=1  Side=Left
  busOut : PMIOPort  Port=2  Side=Right
  accPaxAlight : Outport
  accPaxDemand : Outport  Port=2
  crnVacancy : Outport  Port=3
  paxAlight : Outport  Port=4
  paxDemand : Outport  Port=5
  busIDAfterPaxCal : Outport  Port=6
  newVacancy : Outport  Port=7
  paxBoard : Outport  Port=8
  paxRemain : Outport  Port=9
  paxWait : Outport  Port=10
  intgPaxArr : Outport  Port=11
  intgPaxAlight : Outport  Port=12
  idBusLeave : Outport  Port=13
  wires:
  calcPaxActivThisStop/4(busID) -> busIDAfterPaxCal/1
  calcPaxActivThisStop/1(vacanIn) -> crnVacancy/1
  calcPaxActivThisStop/5(newVacan) -> newVacancy/1
  calcPaxActivThisStop/7(paxRemain) -> paxRemain/1
  paxAlightRate/1 -> integrPaxAlightS1/1(ratePax)
  calcPaxActivThisStop/3(paxArr) -> paxDemand/1
  busDwellThisStop/1(idBusLeave) -> idBusLeave/1
  calcPaxActivThisStop/6(paxBoard) -> paxBoard/1
  calcPaxActivThisStop/9(intgPaxArr) -> intgPaxArr/1
  calcPaxActivThisStop/8(paxWait) -> paxWait/1
  integrPaxArrS1/1(accPax) -> accPaxDemand/1, setPaxAttribThisStop/1
  integrPaxAlightS1/1(accPax) -> accPaxAlight/1, setPaxAttribThisStop/2
  calcPaxActivThisStop/11(dwellTime) -> busDwellThisStop/1(dwellTime)
  calcPaxActivThisStop/10(intgPaxAlight) -> intgPaxAlight/1
  calcPaxActivThisStop/2(paxAlight) -> paxAlight/1
  paxDemandRate/1 -> integrPaxArrS1/1(ratePax)
  connections:
  FIFO Queue9/LConn1 -- busIn/RConn1
  busDwellThisStop/RConn1 -- busOut/RConn1
  setPaxAttribThisStop/RConn1 -- calcPaxActivThisStop/LConn1
  FIFO Queue9/RConn1 -- setPaxAttribThisStop/LConn1
  busDwellThisStop/LConn1 -- calcPaxActivThisStop/RConn1

== system simRouteA_v4_11/chkSchedTimeNormalBusAtCP2 ==
  tTableChkPnt : Inport
  Clock3 : Clock
  FIFO Queue3 : FIFOQueue
  Get Attribute20 : GetAttribute  AttributeName=ID  EvaluatedDefaultAttributeValue={ []}
      settings: OutputPortMap=o1
  Set Attribute7 : SetAttribute  AttributeName=tSchedCP2|timeCP2  AttributeFrom=Signal port|Signal port  AttributeValue=1|1  AttributeTreatAsVector=1|1  EvaluatedAttributeValue={ []; [] }
      settings: InputPortMap=u0,u1
  Subsystem2 : Subsystem  TreatAsAtomicUnit=on
      settings: MinAlgLoopOccurrences=on
  T2E32 : TimedToEventSignal
  T2E33 : TimedToEventSignal
  While Iterator Subsystem : Subsystem  Commented=on  TreatAsAtomicUnit=on
  Conn1 : PMIOPort  Port=1  Side=Left
  Conn2 : PMIOPort  Port=2  Side=Right
  wires:
  tTableChkPnt/1 -> T2E33/1
  T2E33/1 -> Subsystem2/2(tTable)
  Subsystem2/1(schedTime) -> Set Attribute7/1
  Get Attribute20/1 -> Subsystem2/1(ID)
  T2E32/1 -> Set Attribute7/2
  Clock3/1 -> T2E32/1
  connections:
  FIFO Queue3/RConn1 -- Set Attribute7/LConn1
  Conn2/RConn1 -- Set Attribute7/RConn1
  Get Attribute20/LConn1 -- Conn1/RConn1
  Get Attribute20/RConn1 -- FIFO Queue3/LConn1

== system simRouteA_v4_11/chkSchedTimeNormalBusAtCP3 ==
  tTableChkPnt : Inport
  Clock3 : Clock
  FIFO Queue3 : FIFOQueue
  Get Attribute20 : GetAttribute  AttributeName=ID  EvaluatedDefaultAttributeValue={ []}
      settings: OutputPortMap=o1
  Set Attribute7 : SetAttribute  AttributeName=tSchedCP3|timeCP3  AttributeFrom=Signal port|Signal port  AttributeValue=1|1  AttributeTreatAsVector=1|1  EvaluatedAttributeValue={ []; [] }
      settings: InputPortMap=u0,u1
  Subsystem2 : Subsystem  TreatAsAtomicUnit=on
      settings: MinAlgLoopOccurrences=on
  T2E32 : TimedToEventSignal
  T2E33 : TimedToEventSignal
  While Iterator Subsystem : Subsystem  Commented=on  TreatAsAtomicUnit=on
  Conn1 : PMIOPort  Port=1  Side=Left
  Conn2 : PMIOPort  Port=2  Side=Right
  wires:
  tTableChkPnt/1 -> T2E33/1
  T2E33/1 -> Subsystem2/2(tTable)
  Subsystem2/1(schedTime) -> Set Attribute7/1
  Get Attribute20/1 -> Subsystem2/1(ID)
  T2E32/1 -> Set Attribute7/2
  Clock3/1 -> T2E32/1
  connections:
  FIFO Queue3/RConn1 -- Set Attribute7/LConn1
  Conn2/RConn1 -- Set Attribute7/RConn1
  Get Attribute20/LConn1 -- Conn1/RConn1
  Get Attribute20/RConn1 -- FIFO Queue3/LConn1

== system simRouteA_v4_11/chkSchedTimeNormalBusAtCP4 ==
  tTableChkPnt : Inport
  Clock3 : Clock
  FIFO Queue3 : FIFOQueue
  Get Attribute20 : GetAttribute  AttributeName=ID  EvaluatedDefaultAttributeValue={ []}
      settings: OutputPortMap=o1
  Set Attribute7 : SetAttribute  AttributeName=tSchedCP4|timeCP4  AttributeFrom=Signal port|Signal port  AttributeValue=1|1  AttributeTreatAsVector=1|1  EvaluatedAttributeValue={ []; [] }
      settings: InputPortMap=u0,u1
  Subsystem2 : Subsystem  TreatAsAtomicUnit=on
      settings: MinAlgLoopOccurrences=on
  T2E32 : TimedToEventSignal
  T2E33 : TimedToEventSignal
  While Iterator Subsystem : Subsystem  Commented=on  TreatAsAtomicUnit=on
  Conn1 : PMIOPort  Port=1  Side=Left
  Conn2 : PMIOPort  Port=2  Side=Right
  wires:
  tTableChkPnt/1 -> T2E33/1
  T2E33/1 -> Subsystem2/2(tTable)
  Subsystem2/1(schedTime) -> Set Attribute7/1
  Get Attribute20/1 -> Subsystem2/1(ID)
  T2E32/1 -> Set Attribute7/2
  Clock3/1 -> T2E32/1
  connections:
  FIFO Queue3/RConn1 -- Set Attribute7/LConn1
  Conn2/RConn1 -- Set Attribute7/RConn1
  Get Attribute20/LConn1 -- Conn1/RConn1
  Get Attribute20/RConn1 -- FIFO Queue3/LConn1

== system simRouteA_v4_11/holdBusAtCP2 ==
  Get Attribute7 : GetAttribute  AttributeName=ID|tSchedCP2|timeCP2  AttributeMissing=Error|Error|Error  AttributeDefaultValue=1|1|1  AttributeTreatAsVector=1|1|1  AttributeSendTiming=After entity departure|After entity departure|After entity departure  EvaluatedDefaultAttributeValue={ []; []; []}
      settings: OutputPortMap=o1,o2,o3
  HoldMultiBusCP : InfiniteServer  ServiceTimeFrom=Signal port t
  While Iterator Subsystem : Subsystem  Commented=on  TreatAsAtomicUnit=on
  calculateHoldTimeAtCP : Subsystem  TreatAsAtomicUnit=on
  dummyServer1 : SingleServer  ServiceTime=0
  Conn1 : PMIOPort  Port=1  Side=Left
  Conn2 : PMIOPort  Port=2  Side=Right
  idB4CP : Outport
  tSchedCP : Outport  Port=2
  tHoldCP : Outport  Port=3
  wires:
  calculateHoldTimeAtCP/1(tHoldCrnBus) -> tHoldCP/1, HoldMultiBusCP/1
  Get Attribute7/2 -> tSchedCP/1, calculateHoldTimeAtCP/1(crnSchedAtCP)
  Get Attribute7/3 -> calculateHoldTimeAtCP/2(time)
  Get Attribute7/1 -> idB4CP/1
  connections:
  dummyServer1/RConn1 -- HoldMultiBusCP/LConn1
  Get Attribute7/RConn1 -- dummyServer1/LConn1
  Conn1/RConn1 -- Get Attribute7/LConn1
  Conn2/RConn1 -- HoldMultiBusCP/RConn1

== system simRouteA_v4_11/holdBusAtCP3 ==
  Get Attribute7 : GetAttribute  AttributeName=ID|tSchedCP3|timeCP3  AttributeMissing=Error|Error|Error  AttributeDefaultValue=1|1|1  AttributeTreatAsVector=1|1|1  AttributeSendTiming=After entity departure|After entity departure|After entity departure  EvaluatedDefaultAttributeValue={ []; []; []}
      settings: OutputPortMap=o1,o2,o3
  HoldMultiBusCP : InfiniteServer  ServiceTimeFrom=Signal port t
  While Iterator Subsystem : Subsystem  Commented=on  TreatAsAtomicUnit=on
  calculateHoldTimeAtCP : Subsystem  TreatAsAtomicUnit=on
  dummyServer1 : SingleServer  ServiceTime=0
  Conn1 : PMIOPort  Port=1  Side=Left
  Conn2 : PMIOPort  Port=2  Side=Right
  idB4CP : Outport
  tSchedCP : Outport  Port=2
  tHoldCP : Outport  Port=3
  wires:
  calculateHoldTimeAtCP/1(tHoldCrnBus) -> tHoldCP/1, HoldMultiBusCP/1
  Get Attribute7/2 -> tSchedCP/1, calculateHoldTimeAtCP/1(crnSchedAtCP)
  Get Attribute7/3 -> calculateHoldTimeAtCP/2(time)
  Get Attribute7/1 -> idB4CP/1
  connections:
  dummyServer1/RConn1 -- HoldMultiBusCP/LConn1
  Get Attribute7/RConn1 -- dummyServer1/LConn1
  Conn1/RConn1 -- Get Attribute7/LConn1
  Conn2/RConn1 -- HoldMultiBusCP/RConn1

== system simRouteA_v4_11/holdBusAtCP4 ==
  Get Attribute7 : GetAttribute  AttributeName=ID|tSchedCP4|timeCP4  AttributeMissing=Error|Error|Error  AttributeDefaultValue=1|1|1  AttributeTreatAsVector=1|1|1  AttributeSendTiming=After entity departure|After entity departure|After entity departure  EvaluatedDefaultAttributeValue={ []; []; []}
      settings: OutputPortMap=o1,o2,o3
  HoldMultiBusCP : InfiniteServer  ServiceTimeFrom=Signal port t
  While Iterator Subsystem : Subsystem  Commented=on  TreatAsAtomicUnit=on
  calculateHoldTimeAtCP : Subsystem  TreatAsAtomicUnit=on
  dummyServer1 : SingleServer  ServiceTime=0
  Conn1 : PMIOPort  Port=1  Side=Left
  Conn2 : PMIOPort  Port=2  Side=Right
  idB4CP : Outport
  tSchedCP : Outport  Port=2
  tHoldCP : Outport  Port=3
  wires:
  calculateHoldTimeAtCP/1(tHoldCrnBus) -> tHoldCP/1, HoldMultiBusCP/1
  Get Attribute7/2 -> tSchedCP/1, calculateHoldTimeAtCP/1(crnSchedAtCP)
  Get Attribute7/3 -> calculateHoldTimeAtCP/2(time)
  Get Attribute7/1 -> idB4CP/1
  connections:
  dummyServer1/RConn1 -- HoldMultiBusCP/LConn1
  Get Attribute7/RConn1 -- dummyServer1/LConn1
  Conn1/RConn1 -- Get Attribute7/LConn1
  Conn2/RConn1 -- HoldMultiBusCP/RConn1

== system simRouteA_v4_11/inTransitLinkL1 ==
  xtraDelay : Inport
  theoTravTime : Inport  Port=2
  Add : Sum
  Buses being hold on the street : InfiniteServer  ServiceTimeFrom=Signal port t
  Clock2 : Clock
  DummyServer : SingleServer  ServiceTime=0
  FIFO Queue1 : FIFOQueue
  FIFO Queue3 : FIFOQueue
  FIFO Queue9 : FIFOQueue
  Get Attribute : GetAttribute  AttributeName=ID  EvaluatedDefaultAttributeValue={ []}
      settings: OutputPortMap=o1
  Get Attribute5 : GetAttribute  AttributeName=tTrav|time  AttributeMissing=Error|Error  AttributeDefaultValue=1|1  AttributeTreatAsVector=1|1  AttributeSendTiming=After entity departure|After entity departure  EvaluatedDefaultAttributeValue={ []; []}
      settings: OutputPortMap=o1,o2
  Set Attribute3 : SetAttribute  AttributeName=tTrav|time  AttributeFrom=Signal port|Signal port  AttributeValue=1|1  AttributeTreatAsVector=1|1  EvaluatedAttributeValue={ []; [] }
      settings: InputPortMap=u0,u1
  Subsystem2 : Subsystem  TreatAsAtomicUnit=on
  T2E4 : TimedToEventSignal
  busesOutLink : PMIOPort  Port=1  Side=Right
  busesHitTheRoad : PMIOPort  Port=2  Side=Left
  idBusOutLink : Outport
  wires:
  xtraDelay/1 -> Add/1
  theoTravTime/1 -> Add/2
  Add/1 -> Set Attribute3/1
  Get Attribute/1 -> idBusOutLink/1
  Clock2/1 -> T2E4/1
  T2E4/1 -> Set Attribute3/2
  Get Attribute5/1 -> Subsystem2/1(tTrav)
  Get Attribute5/2 -> Subsystem2/2(tDep)
  Subsystem2/1(tTravNew) -> Buses being hold on the street/1
  connections:
  Buses being hold on the street/RConn1 -- FIFO Queue9/LConn1
  FIFO Queue1/LConn1 -- busesHitTheRoad/RConn1
  Get Attribute/RConn1 -- busesOutLink/RConn1
  FIFO Queue9/RConn1 -- Get Attribute/LConn1
  FIFO Queue1/RConn1 -- Set Attribute3/LConn1
  Set Attribute3/RConn1 -- FIFO Queue3/LConn1
  FIFO Queue3/RConn1 -- Get Attribute5/LConn1
  Get Attribute5/RConn1 -- DummyServer/LConn1
  DummyServer/RConn1 -- Buses being hold on the street/LConn1
